simulink model "sgMdl_IO131_Loopback"  (R2024b)
settings: Solver=FixedStepAuto  StartTime=0.0  StopTime=inf  RelTol=1e-3  EnableMultiTasking=on
libraries: speedgoatlib_IO131 x3
Description:
  | IO131 - Analog Loopback
settings Model: sg_rtwmakecfg_data=_sglibc_  ModifiedByFormat=Speedgoat  Creator=Speedgoat  LastModifiedBy=Speedgoat
settings SolverCC: ConcurrentTasks=on  AlgebraicLoopSolver=TrustRegion  PositivePriorityOrder=on  AutoInsertRateTranBlk=on  InsertRTBMode=Never (minimum delay)
settings DataIOCC: SaveFormat=StructureWithTime  ReturnWorkspaceOutputs=off
settings OptimizationCC: BlockReduction=off  OptimizeBlockIOStorage=off  BufferReuse=off  GlobalBufferReuse=off  ExpressionFolding=off  LocalBlockOutputs=off
settings DebuggingCC: TasksWithSamePriorityMsg=none  UnconnectedInputMsg=warning  UnconnectedOutputMsg=warning  UnconnectedLineMsg=warning  SFExecutionAtInitializationDiag=none  ArithmeticOperatorsInVariantConditions=warning
settings HardwareCC: ProdBitPerLong=64  ProdLongLongMode=on  ProdHWDeviceType=Intel->x86-64 (Linux 64)
settings ModelReferenceCC: EnableRefExpFcnMdlSchedulingChecks=on
settings SFSimCC: SimUseLocalCustomCode=off  CustomCodeUndefinedFunction=UseInterfaceOnly
settings RTWCC: Description=Speedgoat Real-Time Target Machine  SystemTargetFile=speedgoat.tlc  TemplateMakefile=slrealtime_default_tmf  RTWUseLocalCustomCode=off  Toolchain=Simulink Real-Time Toolchain  BuildConfiguration=Faster Runs  TargetLang=C++  GPUComputeCapability=3.5  DLArmComputeVersion=19.05
settings CodeAppCC: StateflowObjectComments=on
settings SimulinkRealTimeTargetCC: SubcomponentCodeInterfacePackaging=Reusable function  InstructionSetFMA=off  LogToMDFFile=off  SLRTFileLogMaxRuns=10  UseGCCFastMath=on
settings ConfigComp: CovBoundaryAbsTol=1.0e-5

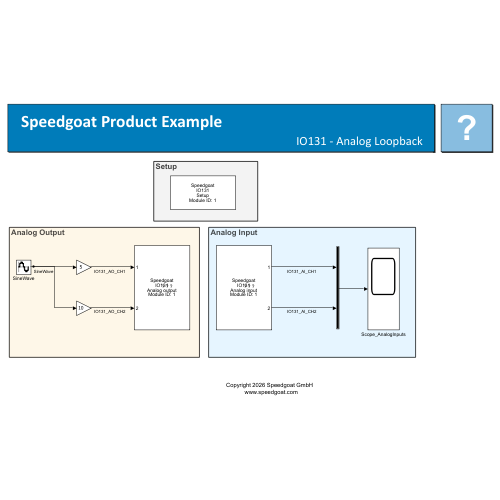
[thumbnail: Simulink's stored preview of the top-level diagram]
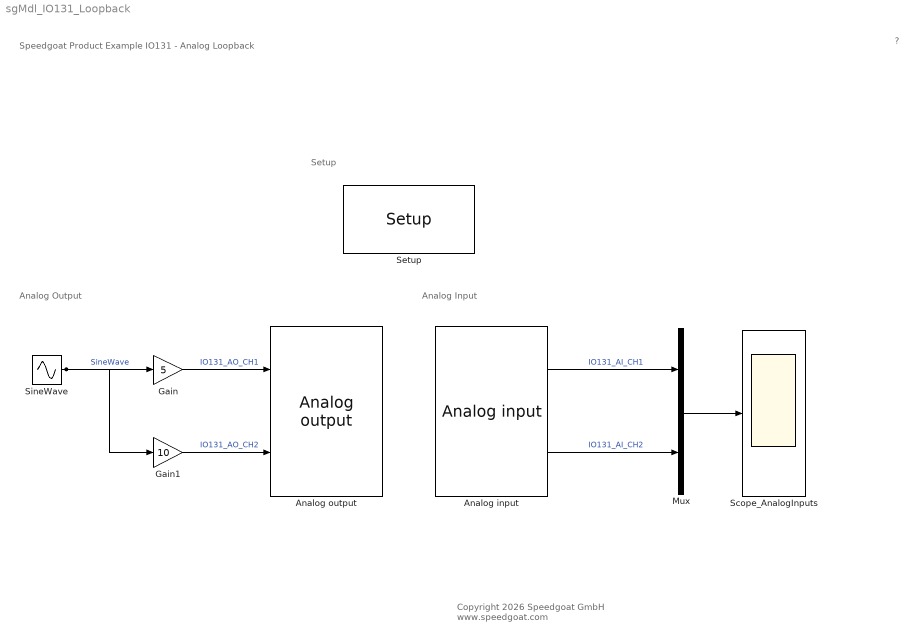
== system sgMdl_IO131_Loopback ==
  note: Setup
  note: Analog Output
  note: Analog Input
  note: Speedgoat Product Example
      | IO131 - Analog Loopback
  note: ?
  note: Copyright 2026 Speedgoat GmbH
      |  www.speedgoat.com
  "Analog input " : speedgoatlib_IO131/Analog input   parModuleId=1  parSampleTime=0.001  parPciSlot=-1  parRange=+-10V  parOversampling=None  parChannels=[1 2]  parContinuousSampling=off  parDmaEn=off  parDmaChannels=All  parDmaConversionTime=100  parDmaFrameSize=128  parBoardType=131  parIsInitialized=on
      settings: SourceProductName=Simulink Real-Time: Speedgoat I/O Blockset
  "Analog output " : speedgoatlib_IO131/Analog output   parModuleId=1  parSampleTime=0.001  parPciSlot=-1  parRange=+-10V  parChannels=[1 2]  parInitValues=[0 0]  parResetValues=[1 1]  parDmaChannels=All  parDmaEn=off  parDmaClkSrc=2  parDmaConversionTime=100  parDmaFrameSize=128  parBoardType=131  parDoInterrupt=on  parLatency=As small as possible  parIsInitialized=on
      settings: SourceProductName=Simulink Real-Time: Speedgoat Library
  Gain : Gain  Gain=5
  Gain1 : Gain  Gain=10
  Mux : Mux  Inputs=2
  Scope_AnalogInputs : Scope
  "Setup " : speedgoatlib_IO131/Setup   parPciSlot=-1  parModuleId=1  parTriggerInitiator=Independent  parAdChannels=[1 2]  parAdRange=+-10V  parAdOversampling=None  parAdContinuousSampling=off  parAdDmaEn=off  parAdDisableCheck=off  parAdDmaChannels=All  parAdSampleClock=100e3  parAdDmaFrameSize=128  parAdSampleTime=0.00128  parDaChannels=[1 2]  parDaRange=+-10V  parDaInitValues=[0]  parDaResetValues=[1]  parDaDmaEn=off  parDaDisableCheck=off  parDaDmaChannels=All  parLatency=As small as possible  parDaSampleClock=100000  parClockLocked=off  parDaDmaFrameSize=128  parDaSampleTime=0.00128  parBoardType=131  parForceRefresh=111[]
      settings: SourceProductName=Simulink Real-Time: Speedgoat Library
  SineWave : Sin  Frequency=2*pi  Samples=50  SampleTime=0.001
  wires:
  Gain1/1 -> "Analog output "/2  "IO131_AO_CH2"
  "Analog input "/1 -> Mux/1  "IO131_AI_CH1"
  SineWave/1 -> Gain1/1, Gain/1  "SineWave"
  Gain/1 -> "Analog output "/1  "IO131_AO_CH1"
  Mux/1 -> Scope_AnalogInputs/1
  "Analog input "/2 -> Mux/2  "IO131_AI_CH2"
